simulink model "fel3"  (R2016a)
settings: Solver=VariableStepAuto  SolverMode=SingleTasking  StartTime=0.0  StopTime=20  RelTol=1e-3
settings Model: Creator=Krisz  LastModifiedBy=Krisz
settings DataIOCC: ReturnWorkspaceOutputs=on
settings DebuggingCC: SFUnexpectedBacktrackingDiag=error  SFNoUnconditionalDefaultTransitionDiag=error
settings SFSimCC: SimUseLocalCustomCode=on
settings RTWCC: RTWUseLocalCustomCode=on
settings GRTTargetCC: TargetLangStandard=C99 (ISO)
settings ConfigComp: CovMetricSettings=dwe  CovSaveCumulativeToWorkspaceVar=off  CovSaveSingleToWorkspaceVar=off  CovExternalEMLEnable=on

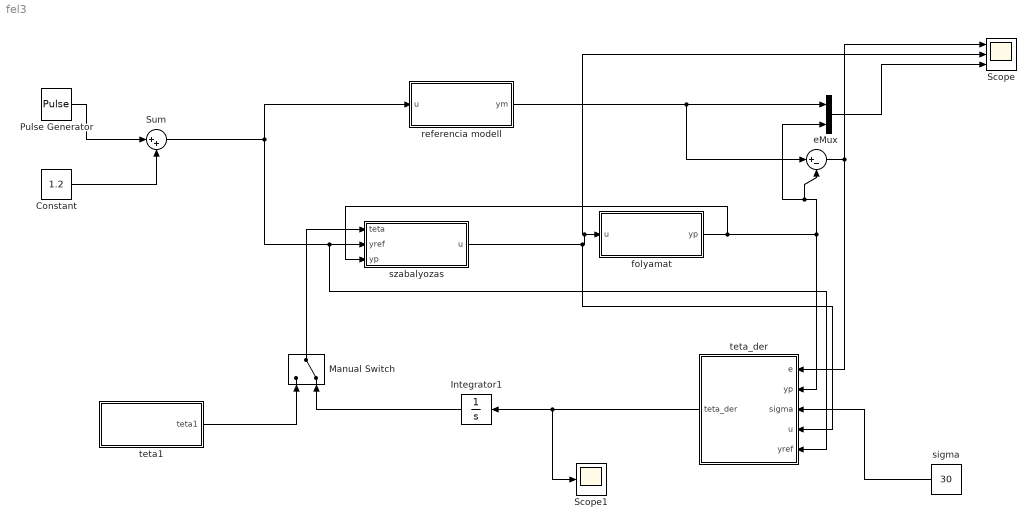
== system fel3 ==
  Constant : Constant  Value=1.2
  Integrator1 : Integrator  InitialCondition=50  LimitOutput=on  UpperSaturationLimit=120  LowerSaturationLimit=1
  Manual Switch : ManualSwitch  CurrentSetting=0
  Mux : Mux  Inputs=2
  Pulse Generator : DiscretePulseGenerator  PulseType=Time based  Period=1  PulseWidth=50
  Scope : Scope  NumInputPorts=3
  Scope1 : Scope
  Sum : Sum  Inputs=|++
  e : Sum  Inputs=|+-
  folyamat : Subsystem
  referencia modell : Subsystem
  sigma : Constant  Value=30
  szabalyozas : Subsystem
  teta1 : Subsystem
  teta_der : Subsystem
  wires:
  sigma/1 -> teta_der/3(sigma)
  folyamat/1(yp) -> szabalyozas/3(yp), teta_der/2(yp), Mux/2, e/2
  Mux/1 -> Scope/3
  Manual Switch/1 -> szabalyozas/1(teta)
  teta1/1(teta1) -> Manual Switch/1
  referencia modell/1(ym) -> Mux/1, e/1
  szabalyozas/1(u) -> teta_der/4(u), folyamat/1(u), Scope/2
  e/1 -> teta_der/1(e), Scope/1
  teta_der/1(teta_der) -> Integrator1/1, Scope1/1
  Pulse Generator/1 -> Sum/1
  Constant/1 -> Sum/2
  Sum/1 -> teta_der/5(yref), szabalyozas/2(yref), referencia modell/1(u)
  Integrator1/1 -> Manual Switch/2

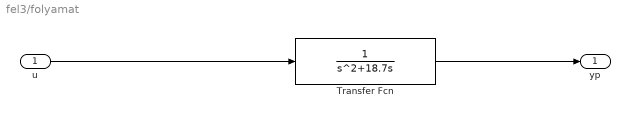
== system fel3/folyamat ==
  u : Inport
  Transfer Fcn : TransferFcn  Denominator=[1 18.7 0]
  yp : Outport
  wires:
  u/1 -> Transfer Fcn/1
  Transfer Fcn/1 -> yp/1

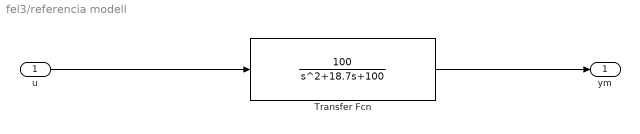
== system fel3/referencia modell ==
  u : Inport
  Transfer Fcn : TransferFcn  Numerator=[100]  Denominator=[1 18.7 100]
  ym : Outport
  wires:
  u/1 -> Transfer Fcn/1
  Transfer Fcn/1 -> ym/1

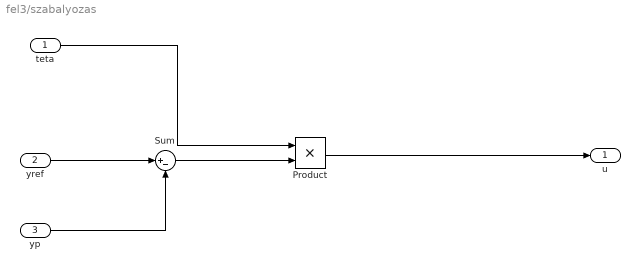
== system fel3/szabalyozas ==
  teta : Inport
  yref : Inport  Port=2
  yp : Inport  Port=3
  Product : Product
  Sum : Sum  Inputs=|+-
  u : Outport
  wires:
  yref/1 -> Sum/1
  yp/1 -> Sum/2
  teta/1 -> Product/1
  Sum/1 -> Product/2
  Product/1 -> u/1

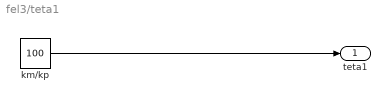
== system fel3/teta1 ==
  km/kp : Constant  Value=100
  teta1 : Outport
  wires:
  km/kp/1 -> teta1/1

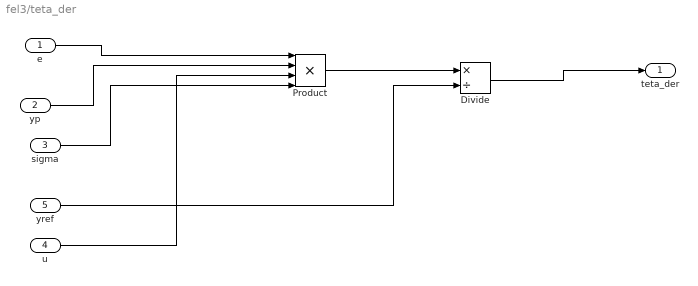
== system fel3/teta_der ==
  e : Inport
  yp : Inport  Port=2
  sigma : Inport  Port=3
  u : Inport  Port=4
  yref : Inport  Port=5
  Divide : Product  Inputs=*/
  Product : Product  Inputs=4
  teta_der : Outport
  wires:
  e/1 -> Product/1
  yp/1 -> Product/2
  sigma/1 -> Product/4
  u/1 -> Product/3
  Product/1 -> Divide/1
  Divide/1 -> teta_der/1
  yref/1 -> Divide/2
